simulink model "Induction_Motor_Ex"  (R2022a)
settings: Solver=VariableStepAuto  StartTime=0.0  StopTime=1  MaxStep=1e-4  RelTol=1e-9
values from neighbouring files (symbols this model uses):
  A = [-1/tau_sigma            0     (R_r * L_m)/(sigma * L_r^2 * L_s) (p * w_me * L_m)/(sigma * L_r * L_s) ... (first row only)    [Induction_Motor_Init_Ex.m]
  A_d = expm(A*T_s)    [Induction_Motor_Init_Ex.m]
  Akf = [Akf;A_d^ii]    [Compute_Akf_Bkf.m]
  B = [1/(sigma * L_s)               0 ... (first row only)    [Induction_Motor_Init_Ex.m]
  B_d = inv(A)*(A_d-eye(4))*B    [Induction_Motor_Init_Ex.m]
  Bkf = [Bkf;Bkf_line]    [Compute_Akf_Bkf.m]
  C = [1 0 0 0 ... (first row only)    [Induction_Motor_Init_Ex.m]
  C_d = C    [Induction_Motor_Init_Ex.m]
  Ckf = blkdiag(Ckf, C_new)    [Compute_D_cal_E_cal_Ckf.m]
  D_cal = [D_cal; D_cal_line;]    [Compute_D_cal_E_cal_Ckf.m]
  E_cal = [E_cal; zeros(m, m)]    [Compute_D_cal_E_cal_Ckf.m]
  i_alphabeta_0 = i_dq_ss    [Induction_Motor_Init_Ex.m]
  K = P*C_d'*inv(C_d*P*C_d'+N)    [Induction_Motor_Init_Ex.m]
  kf = 2    [Induction_Motor_Init_Ex.m]
  Omega_u = [Omega_u;omega_u]    [Compute_constraints.m]
  Omega_x = [Omega_x;omega_x]    [Compute_constraints.m]
  psi_alphabeta_0 = psi_dq_ss    [Induction_Motor_Init_Ex.m]
  Qkf = blkdiag(Qkf,Q)    [Compute_Qkf_Rkf.m]
  Rkf = blkdiag(Rkf,R)    [Compute_Qkf_Rkf.m]
  T_s = 100e-6    (= 0.0001)    [Induction_Motor_Init_Ex.m]
  W_cal_u = blkdiag(W_cal_u,W_u)    [Compute_constraints.m]
  W_cal_x = blkdiag(W_cal_x,W_x)    [Compute_constraints.m]
  w_el = 50  * 2 * pi    (= 314.159265359)    [Induction_Motor_Init_Ex.m]
  x0 = zeros(4,1)    [Induction_Motor_Init_Ex.m]
settings Model: Creator=mschenke  LastModifiedBy=Abdur Rafay
settings SolverCC: AlgebraicLoopSolver=TrustRegion
settings DebuggingCC: UnconnectedInputMsg=warning  UnconnectedOutputMsg=warning  UnconnectedLineMsg=warning
settings SFSimCC: CustomCodeUndefinedFunction=UseInterfaceOnly

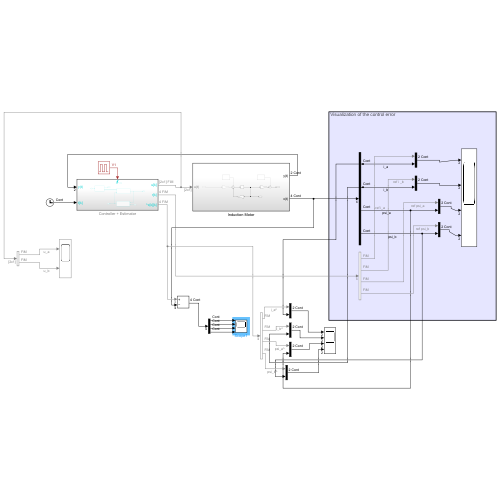
[thumbnail: Simulink's stored preview of the top-level diagram]
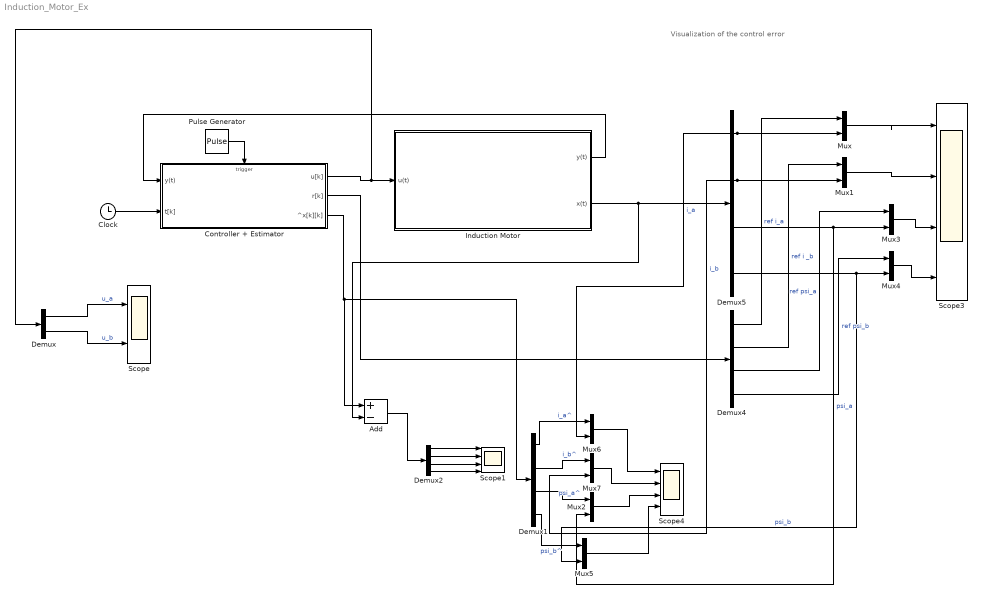
== system Induction_Motor_Ex ==
  note: Visualization of the control error
  Add : Sum  Inputs=+-
  Clock : Clock
  Controller + Estimator : Subsystem
  Demux : Demux  Outputs=2
  Demux{1..2,4..5} (4 alike) : Demux
  Induction Motor : Subsystem
  Mux{,1..7} (8 alike) : Mux  Inputs=2
  Pulse Generator : DiscretePulseGenerator  PulseType=Time based  Period=T_s  PulseWidth=5
  Scope : Scope  NumInputPorts=2
  Scope1 : Scope  NumInputPorts=4
  Scope3 : Scope  NumInputPorts=4
  Scope4 : Scope  NumInputPorts=4
  wires:
  Pulse Generator/1 -> Controller + Estimator/Trigger
  Induction Motor/1(y(t)) -> Controller + Estimator/1(y(t))
  Induction Motor/2(x(t)) -> Add/2, Demux5/1
  Controller + Estimator/1(u[k]) -> Demux/1, Induction Motor/1(u(t))
  Controller + Estimator/2(r[k]) -> Demux4/1
  Clock/1 -> Controller + Estimator/2(t[k])
  Demux4/1 -> Mux/1  "ref i_a"
  Demux5/1 -> Mux6/2, Mux/2  "i_a"
  Demux4/2 -> Mux1/1  "ref i _b"
  Demux5/2 -> Mux7/2, Mux1/2  "i_b"
  Demux4/3 -> Mux3/1  "ref psi_a"
  Demux5/3 -> Mux2/2, Mux3/2  "psi_a"
  Demux4/4 -> Mux4/1  "ref psi_b"
  Demux5/4 -> Mux5/2, Mux4/2  "psi_b"
  Mux5/1 -> Scope4/4
  Demux1/4 -> Mux5/1  "psi_b^"
  Demux1/3 -> Mux2/1  "psi_a^"
  Demux1/2 -> Mux7/1  "i_b^"
  Demux1/1 -> Mux6/1  "i_a^"
  Controller + Estimator/3(^x[k][k]) -> Add/1, Demux1/1
  Demux/1 -> Scope/1  "u_a"
  Demux/2 -> Scope/2  "u_b"
  Mux2/1 -> Scope4/3
  Mux6/1 -> Scope4/1
  Mux7/1 -> Scope4/2
  Mux3/1 -> Scope3/3
  Mux4/1 -> Scope3/4
  Mux/1 -> Scope3/1
  Mux1/1 -> Scope3/2
  Add/1 -> Demux2/1
  Demux2/1 -> Scope1/1
  Demux2/2 -> Scope1/2
  Demux2/3 -> Scope1/3
  Demux2/4 -> Scope1/4

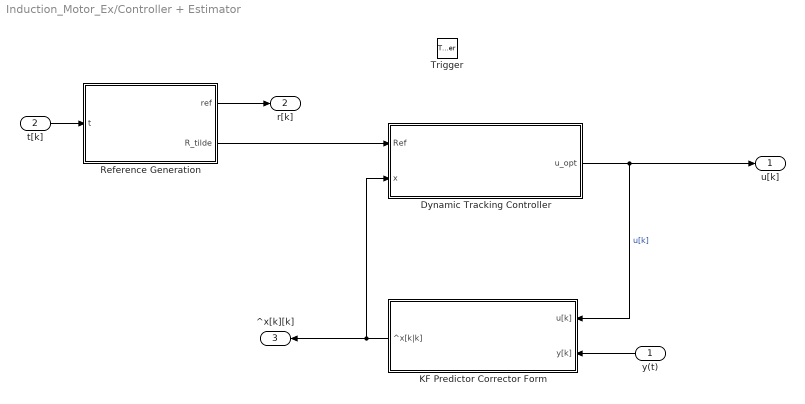
== system Induction_Motor_Ex/Controller + Estimator ==
  y(t) : Inport
  t[k] : Inport  Port=2
  Trigger : TriggerPort  VariantControl=(inherit)  PortDimensions=1
  Dynamic Tracking Controller : MATLAB Function  TreatAsAtomicUnit=on
  KF Predictor Corrector Form : Subsystem
  Reference Generation : MATLAB Function  TreatAsAtomicUnit=on
  u[k] : Outport  VectorParamsAs1DForOutWhenUnconnected=off
  r[k] : Outport  Port=2  VectorParamsAs1DForOutWhenUnconnected=off
  ^x[k][k] : Outport  Port=3  VectorParamsAs1DForOutWhenUnconnected=off
  wires:
  KF Predictor Corrector Form/1(^x[k|k]) -> ^x[k][k]/1, Dynamic Tracking Controller/2(x)
  Reference Generation/2(R_tilde) -> Dynamic Tracking Controller/1(Ref)
  Dynamic Tracking Controller/1(u_opt) -> KF Predictor Corrector Form/1(u[k]), u[k]/1  "u[k]"
  t[k]/1 -> Reference Generation/1(t)
  y(t)/1 -> KF Predictor Corrector Form/2(y[k])
  Reference Generation/1(ref) -> r[k]/1

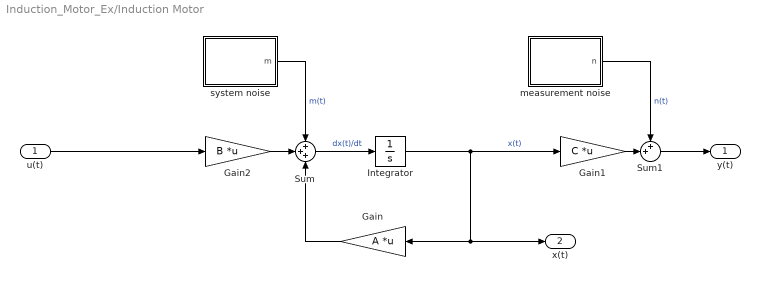
== system Induction_Motor_Ex/Induction Motor ==
  u(t) : Inport
  Gain : Gain  Gain=A  Multiplication=Matrix(K*u) (u vector)
  Gain1 : Gain  Gain=C  Multiplication=Matrix(K*u) (u vector)
  Gain2 : Gain  Gain=B  Multiplication=Matrix(K*u) (u vector)
  Integrator : Integrator  InitialCondition=x0
  Sum : Sum  Inputs=+++
  Sum1 : Sum  Inputs=++|
  measurement noise : MATLAB Function  TreatAsAtomicUnit=on
  system noise : MATLAB Function  TreatAsAtomicUnit=on
  y(t) : Outport
  x(t) : Outport  Port=2
  wires:
  Sum/1 -> Integrator/1  "dx(t)/dt"
  Integrator/1 -> x(t)/1, Gain/1, Gain1/1  "x(t)"
  u(t)/1 -> Gain2/1
  Gain/1 -> Sum/3
  Gain2/1 -> Sum/2
  Gain1/1 -> Sum1/2
  Sum1/1 -> y(t)/1
  system noise/1(m) -> Sum/1  "m(t)"
  measurement noise/1(n) -> Sum1/1  "n(t)"

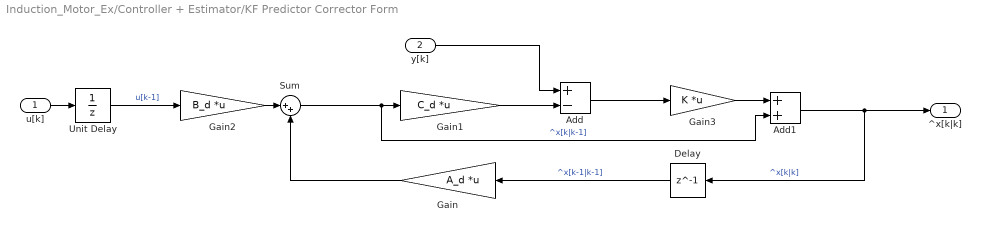
== system Induction_Motor_Ex/Controller + Estimator/KF Predictor Corrector Form ==
  u[k] : Inport
  y[k] : Inport  Port=2
  Add : Sum  Inputs=+-
  Add1 : Sum
  Delay : Delay  DelayLength=1  InitialCondition=x0
  Gain : Gain  Gain=A_d  Multiplication=Matrix(K*u) (u vector)
  Gain1 : Gain  Gain=C_d  Multiplication=Matrix(K*u) (u vector)
  Gain2 : Gain  Gain=B_d  Multiplication=Matrix(K*u) (u vector)
  Gain3 : Gain  Gain=K  Multiplication=Matrix(K*u) (u vector)
  Sum : Sum  Inputs=|++
  Unit Delay : UnitDelay  SampleTime=-1  HasFrameUpgradeWarning=on
  ^x[k|k] : Outport
  wires:
  u[k]/1 -> Unit Delay/1
  y[k]/1 -> Add/1
  Unit Delay/1 -> Gain2/1  "u[k-1]"
  Add1/1 -> ^x[k|k]/1, Delay/1  "^x[k|k]"
  Gain3/1 -> Add1/1
  Add/1 -> Gain3/1
  Gain1/1 -> Add/2
  Gain2/1 -> Sum/1
  Gain/1 -> Sum/2
  Delay/1 -> Gain/1  "^x[k-1|k-1]"
  Sum/1 -> Add1/2, Gain1/1  "^x[k|k-1]"

== matlab function Induction_Motor_Ex/Induction Motor/measurement noise ==
  data: n output
function n = fcn()
n=randn(2,1).*sqrt([1e-3 1e-3]');

== matlab function Induction_Motor_Ex/Induction Motor/system noise ==
  data: m output
function m = fcn()
m=randn(4,1).*sqrt([1e-5 1e-5 1e-5 1e-5]');

== matlab function Induction_Motor_Ex/Controller + Estimator/Reference Generation ==
  data: t input; ref output; psi_alphabeta_0 parameter; R_tilde output size=1000; T_s parameter; kf parameter; w_el parameter; i_alphabeta_0 parameter
function [ref, R_tilde]= fcn(t,psi_alphabeta_0, T_s, kf, w_el, i_alphabeta_0)

ref = [[cos(t*w_el)  -sin(t*w_el);
        sin(t*w_el)   cos(t*w_el)]*i_alphabeta_0;
       [cos(t*w_el)  -sin(t*w_el);
        sin(t*w_el)   cos(t*w_el)]*psi_alphabeta_0];

R_tilde = ref;

for ii = 1:kf
    R_tilde = [R_tilde;
               [cos((t + ii * T_s)*w_el)   -sin((t + ii * T_s)*w_el);
                sin((t + ii * T_s)*w_el)    cos((t + ii * T_s)*w_el)]*i_alphabeta_0;
               [cos((t + ii * T_s)*w_el)   -sin((t + ii * T_s)*w_el);
                sin((t + ii * T_s)*w_el)    cos((t + ii * T_s)*w_el)]*psi_alphabeta_0];
end

end

== matlab function Induction_Motor_Ex/Controller + Estimator/Dynamic Tracking Controller ==
  data: Ref input; x input; u_opt output size=[2 1]; Akf parameter; Bkf parameter; Ckf parameter; Qkf parameter; Rkf parameter; E_cal parameter; D_cal parameter; W_cal_x parameter; W_cal_u parameter; Omega_x parameter; Omega_u parameter
function u_opt = fcn(Ref, x, Akf, Bkf, Ckf, Qkf, Rkf, E_cal, D_cal, W_cal_x, W_cal_u, Omega_x, Omega_u)
coder.extrinsic('quadprog')

persistent u_old

if isempty(u_old)
    u_old = zeros(2, 1);
    u_opt = zeros(2, 1); 
end

% Solution of the QP


H = 2 * (Bkf' * Ckf' * Qkf * Ckf * Bkf + (eye(length(D_cal)) - D_cal)' * Rkf * (eye(length(D_cal)) - D_cal));
f = 2 * (x' * Akf' * Ckf' * Qkf * Ckf * Bkf - Ref' * Qkf * Ckf * Bkf - u_old' * E_cal' * Rkf * (eye(length(D_cal)) - D_cal))';
G = [W_cal_x * Bkf; W_cal_u;];
e = [Omega_x - W_cal_x * Akf * x; Omega_u;];

z_opt = quadprog(H, f, G, e);
u_opt = z_opt(1:2);
u_old = u_opt;
end
